simulink model "continuoustest"  (R2016a)
settings: Solver=VariableStepAuto  StartTime=0.0  StopTime=10000  RelTol=1e-2
values from neighbouring files (symbols this model uses):
  c = 5.373169834e-7    (= 5.373169834e-07)    [comparison.m]    (also in heating.m; heating_PID.m; heating_eggs.m; heating_new.m)
  k = (1.256e-5*m^2 - 0.00008313*m + 0.0002086) + v*(1.77e-5*m^2 - 0.0001243.*m + 0.0002314)/6    [k_exp.m]    (also in main_plot.m = [0.0001331, 0.000104, 0.0001246, 0.00008305, 0.0001337, 0.00; new_open_loop.m = 0.00019; open_loop.m = 0.00019; statespacetest_tonja.m = k_exp(m,6))
  m = 2    [comparison.m]    (also in model.m; new_open_loop.m = 3; open_loop.m; statespacetest_tonja.m)
libraries: simulink x2
settings Model: Creator=tonie  LastModifiedBy=tonie

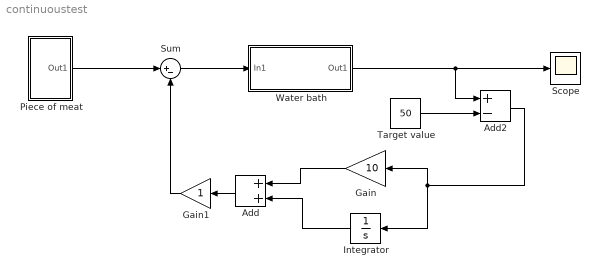
== system continuoustest ==
  Add : Sum
  Add2 : Sum  Inputs=+-
  Gain : Gain  Gain=10
  Gain1 : Gain
  Integrator : Integrator
  Piece of meat : Subsystem
  Scope : Scope
  Sum : Sum  Inputs=|+-
  Target value : Constant  Value=50
  Water bath : Subsystem
  wires:
  Sum/1 -> Water bath/1(In1)
  Gain/1 -> Add/1
  Water bath/1(Out1) -> Add2/1, Scope/1
  Integrator/1 -> Add/2
  Add/1 -> Gain1/1
  Gain1/1 -> Sum/2
  Add2/1 -> Integrator/1, Gain/1
  Target value/1 -> Add2/2
  Piece of meat/1(Out1) -> Sum/1

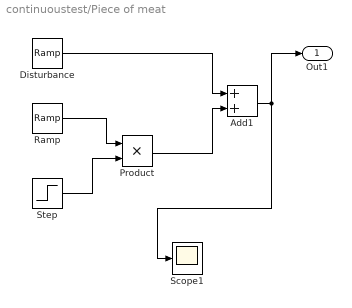
== system continuoustest/Piece of meat ==
  Add1 : Sum
  Disturbance : simulink/Sources/Ramp  slope=0.01  start=0  X0=-30
  Product : Product
  Ramp : simulink/Sources/Ramp  slope=-0.01  start=0  X0=80
  Scope1 : Scope
  Step : Step  Time=8000  SampleTime=0
  Out1 : Outport
  wires:
  Product/1 -> Add1/2
  Step/1 -> Product/2
  Ramp/1 -> Product/1
  Disturbance/1 -> Add1/1
  Add1/1 -> Out1/1, Scope1/1

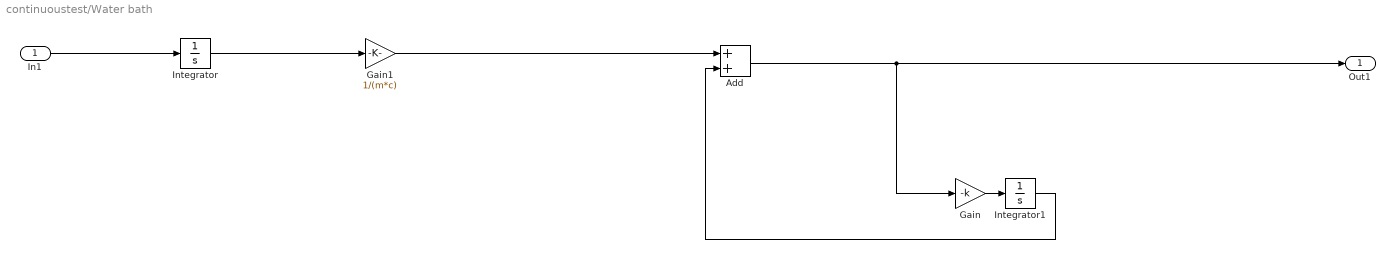
== system continuoustest/Water bath ==
  In1 : Inport
  Add : Sum
  Gain : Gain  Gain=-k
  Gain1 : Gain  Gain=1/(m*c)
  Integrator : Integrator
  Integrator1 : Integrator
  Out1 : Outport
  wires:
  In1/1 -> Integrator/1
  Integrator/1 -> Gain1/1
  Gain1/1 -> Add/1
  Add/1 -> Gain/1, Out1/1
  Gain/1 -> Integrator1/1
  Integrator1/1 -> Add/2
